simulink model "verify_relFlowCoeff2qua_mdl"  (R2016b)
settings: Solver=VariableStepDiscrete  StartTime=0.0  StopTime=20  MaxStep=0.1  RelTol=1e-3  EnableMultiTasking=on
libraries: carnot x2, simulink x1
settings Model: Creator=drhf  LastModifiedBy=drhf
settings DataIOCC: LimitDataPoints=on  SaveFormat=Array
settings OptimizationCC: ExpressionDepthLimit=2147483647  LifeSpan=inf
settings DebuggingCC: UnderspecifiedInitializationDetection=Classic  MergeDetectMultiDrivingBlocksExec=none  SolverPrmCheckMsg=warning  StateNameClashWarn=warning  SFUnexpectedBacktrackingDiag=warning  SFNoUnconditionalDefaultTransitionDiag=warning  SFExecutionAtInitializationDiag=none
settings HardwareCC: ProdBitPerPointer=32  ProdBitPerSizeT=32  ProdBitPerPtrDiffT=32  ProdLargestAtomicFloat=None  ProdIntDivRoundTo=Undefined  ProdEndianess=Unspecified  ProdWordSize=32  ProdHWDeviceType=32-bit Generic
settings ModelReferenceCC: PropagateSignalLabelsOutOfModel=off
settings GRTTargetCC: TargetLangStandard=C89/C90 (ANSI)  GeneratePreprocessorConditionals=Disable all  CombineOutputUpdateFcns=off  GRTInterface=on
settings ConfigComp: CovMetricSettings=dw  CovHtmlReporting=on  CovSaveCumulativeToWorkspaceVar=on  CovSaveSingleToWorkspaceVar=on  CovExternalEMLEnable=off

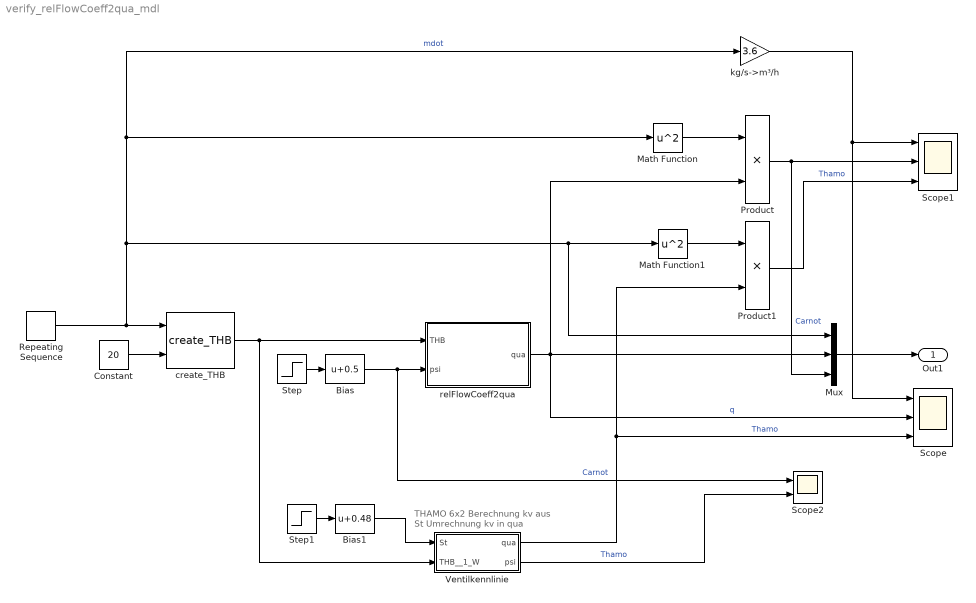
== system verify_relFlowCoeff2qua_mdl ==
  note: THAMO 6x2
      |
      |
      |
      |
      |
      |
      | Berechnung kv aus St
      | Umrechnung kv in qua
  Bias : Bias  Bias=0.5
  Bias1 : Bias  Bias=0.48
  Constant : Constant  Value=20
  Math Function : Math  Operator=square  SaturateOnIntegerOverflow=on
  Math Function1 : Math  Operator=square  SaturateOnIntegerOverflow=on
  Mux : Mux  Inputs=3
  Product : Product
  Product1 : Product
  Repeating Sequence : simulink/Sources/Repeating Sequence  rep_seq_t=[0 10]  rep_seq_y=[0 1.6/3.6]
  Scope : Scope  NumInputPorts=3
  Scope1 : Scope  NumInputPorts=3
  Scope2 : Scope  NumInputPorts=2
  Step : Step  Time=10  After=0.5  SampleTime=0
  Step1 : Step  Time=10  After=0.52  SampleTime=0
  Ventilkennlinie : Subsystem
  create_THB : carnot/Source/Simple/create_THB  p=1e5  fluid=Water  mix=0  mix2=0  mix3=0  dia=0.02  hgt=0  mID=Pressure Drop from Massflow
  kg/s->m³/h : Gain  Gain=3.6
  relFlowCoeff2qua : Subsystem  mask{kvs=1.6}
      mask prompts: kvs "Flow coefficient of open valve (Kvs) in m³/h"
      mask TypeOptions kvs: Kvs/Gain
      mask Display: disp('rel\nFlow Coeff\nto qua')
  Out1 : Outport  SampleTime=1
  wires:
  Repeating Sequence/1 -> Math Function/1, kg/s->m³/h/1, Mux/1, Math Function1/1, create_THB/1  "mdot"
  Constant/1 -> create_THB/2
  relFlowCoeff2qua/1(qua) -> Scope/2, Mux/2, Product/2  "q"
  create_THB/1 -> relFlowCoeff2qua/1(THB), Ventilkennlinie/2(THB__1_W)
  Ventilkennlinie/1(qua) -> Scope/3, Product1/2  "Thamo"
  Ventilkennlinie/2(psi) -> Scope2/2  "Thamo"
  Math Function/1 -> Product/1
  Math Function1/1 -> Product1/1
  Product/1 -> Mux/3, Scope1/2  "Carnot"
  Product1/1 -> Scope1/3  "Thamo"
  Mux/1 -> Out1/1
  kg/s->m³/h/1 -> Scope/1, Scope1/1
  Step/1 -> Bias/1
  Bias/1 -> Scope2/1, relFlowCoeff2qua/2(psi)  "Carnot"
  Step1/1 -> Bias1/1
  Bias1/1 -> Ventilkennlinie/1(St)

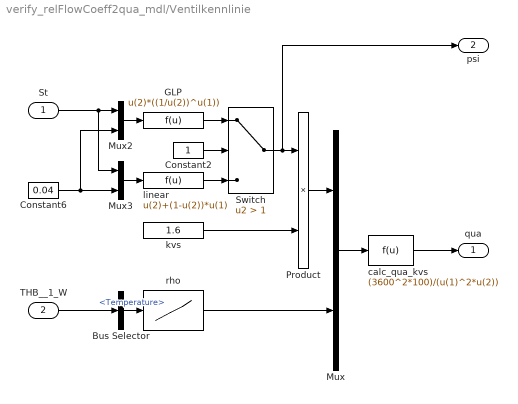
== system verify_relFlowCoeff2qua_mdl/Ventilkennlinie ==
  St : Inport
  THB__1_W : Inport  Port=2
  Bus Selector : BusSelector  OutputSignals=Temperature
  Constant2 : Constant
  Constant6 : Constant  Value=0.04
  GLP : Fcn  Expr=u(2)*((1/u(2))^u(1))
  Mux : Mux  Inputs=2
  Mux2 : Mux  Inputs=2
  Mux3 : Mux  Inputs=2
  Product : Product
  Switch : Switch  Criteria=u2 > Threshold  Threshold=1
  calc_qua_kvs : Fcn  Expr=(3600^2*100)/(u(1)^2*u(2))
  kvs : Constant  Value=1.6
  linear : Fcn  Expr=u(2)+(1-u(2))*u(1)
  rho : Lookup_n-D  NumberOfTableDimensions=1  BreakpointsForDimension1=[0,10,20,30,40,50,60,70,80,90,100]  Table=[999.84,999.7,998.2,995.64,992.21,988.03,983.19,977.76,971.79,965.3,958.35]  InternalRulePriority=Speed  RndMeth=Simplest  InputSameDT=on
  qua : Outport
  psi : Outport  Port=2
  wires:
  Bus Selector/1 -> rho/1  "<Temperature>"
  St/1 -> Mux2/1, Mux3/1
  linear/1 -> Switch/3
  Mux2/1 -> GLP/1
  Mux3/1 -> linear/1
  Constant6/1 -> Mux2/2, Mux3/2
  kvs/1 -> Product/2
  Switch/1 -> psi/1, Product/1
  Constant2/1 -> Switch/2
  GLP/1 -> Switch/1
  THB__1_W/1 -> Bus Selector/1
  calc_qua_kvs/1 -> qua/1
  Mux/1 -> calc_qua_kvs/1
  Product/1 -> Mux/1
  rho/1 -> Mux/2

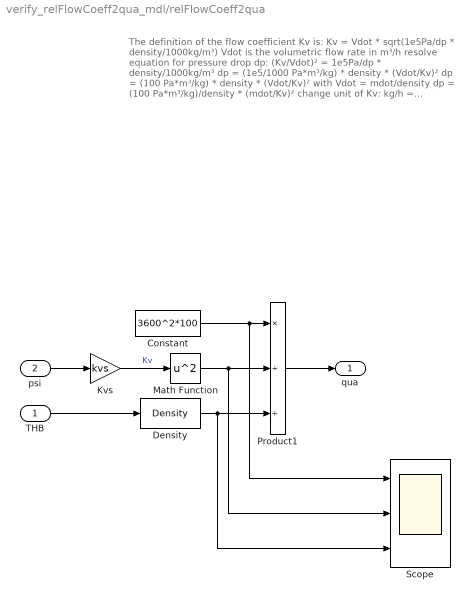
== system verify_relFlowCoeff2qua_mdl/relFlowCoeff2qua ==
  note: The definition of the flow coefficient Kv is:
      | Kv = Vdot * sqrt(1e5Pa/dp * density/1000kg/m³)
      | Vdot is the volumetric flow rate in m³/h
      | resolve equation for pressure drop dp:
      | (Kv/Vdot)² = 1e5Pa/dp * density/1000kg/m³
      | dp = (1e5/1000 Pa*m³/kg) * density * (Vdot/Kv)²
      | dp = (100 Pa*m³/kg) * density * (Vdot/Kv)²
      | with Vdot = mdot/density
      | dp = (100 Pa*m³/kg)/density * (mdot/Kv)²
      | change unit of Kv: kg/h = kg/(3600s)
      | dp = (100 Pa*m³/kg) * (3600 s/h)² / density * (mdot/Kv)²
      | Carnot equation: dp = qua * mdot²
      | qua = (100 Pa*m³/kg) * (3600 s/h)² / (density*Kv²)
  THB : Inport
  psi : Inport  Port=2
  Constant : Constant  Value=3600^2*100
  Density : carnot/Basic/Material_Properties/Density  VariantControl=CarlibClassic  INPUTARGUMENTS=THB  DEBUGLEVEL=DEBUGLEVEL  MAXTOTALWARNINGS=inf  MAXCONSECUTIVEWARNINGS=inf  WRITETOFILE=0  FILENAME='errors.txt'
  Kvs : Gain  Gain=kvs
  Math Function : Math  Operator=square  SaturateOnIntegerOverflow=on
  Product1 : Product  Inputs=*//
  Scope : Scope  NumInputPorts=3
  qua : Outport
  wires:
  THB/1 -> Density/1
  Density/1 -> Scope/3, Product1/3
  Math Function/1 -> Scope/2, Product1/2
  Product1/1 -> qua/1
  Constant/1 -> Scope/1, Product1/1
  psi/1 -> Kvs/1
  Kvs/1 -> Math Function/1  "Kv"
